simulink model "uvms"  (Simulink 7.9)
settings: Solver=ode45  StartTime=0.0  StopTime=10.0  RelTol=1e-3
settings Model: Creator=simena  LastModifiedBy=simena

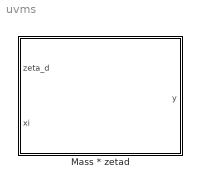
== system uvms ==
  Mass * zetad : MATLAB Function  TreatAsAtomicUnit=on

== matlab function Mass * zetad ==
  data: zeta_d input double; y output double; xi input double
function y = M_zetad(zeta_d,xi)
%#codegen

a=fcn(2);

y=2;


end
